simulink model "Trans_model"  (R2020b)
settings: Solver=VariableStepAuto  StartTime=0.0  StopTime=10.0  RelTol=1e-3
libraries: fl_lib x3, nesl_utility x3, ee_lib x2, powerlib_meascontrol x1, simulink x1
settings Model: Creator=1  LastModifiedBy=1

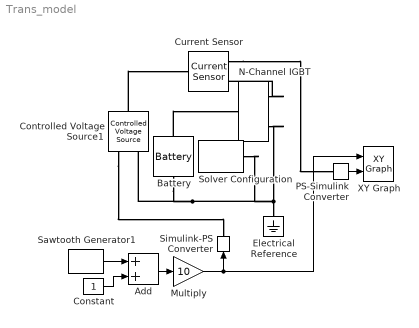
== system Trans_model ==
  Add : Sum
  Battery : ee_lib/Sources/Battery  Vnom=15 V  prm_dir=1  R1_dis=2 Ohm  R1_ch=2 Ohm  R1=1 Ohm  prm_AH=1  AH=50 hr*A  V1=11.5 V  AH1=25 hr*A  prm_R2=1  R2=2000 Ohm  prm_dyn=1  Rp1=0.005 Ohm  tau1=30 s  Rp2=0.005 Ohm  tau2=30 s  Rp3=0.005 Ohm  tau3=30 s  Rp4=0.005 Ohm  tau4=30 s  Rp5=0.005 Ohm  tau5=30 s  prm_fade=1  N_fade=100  AH_fade=45 hr*A  R1_fade=2.02 Ohm  R1_ch_fade=2.02 Ohm  V1_fade=10.35 V  i_specify=off  i_priority=None  i=0 A  i_nominal_specify=off  i_nominal_unit=A  i_nominal_value=1  v_specify=off  v_priority=Low  v=6 V  v_nominal_specify=off  v_nominal_unit=V  v_nominal_value=1  charge_specify=off  charge_priority=High  charge=50 hr*A  charge_nominal_specify=off  charge_nominal_unit=hr*A  charge_nominal_value=1  num_cycles_specify=off  num_cycles_priority=High  num_cycles=0  num_cycles_nominal_specify=off  num_cycles_nominal_unit=1  num_cycles_nominal_value=1  thermal_mass=30000 J/K  Tmeas=298.15 K  Vnom_T2=12 V  R1_T2=2.2 Ohm  R1_T2_dis=2.2 Ohm  R1_T2_ch=2.2 Ohm  V1_T2=11.4 V  R2_T2=2200 Ohm  Rp1_T2=0.005 Ohm  tau1_T2=30 s  Rp2_T2=0.005 Ohm  tau2_T2=30 s  Rp3_T2=0.005 Ohm  tau3_T2=30 s  Rp4_T2=0.005 Ohm  tau4_T2=30 s  Rp5_T2=0.005 Ohm  tau5_T2=30 s  Tmeas2=273.15 K  temperature_specify=off  temperature_priority=High  temperature=298.15 K  temperature_nominal_specify=off  temperature_nominal_unit=K  temperature_nominal_value=1
  Constant : Constant
  Controlled Voltage Source1 : fl_lib/Electrical/Electrical Sources/Controlled Voltage Source
  Current Sensor : fl_lib/Electrical/Electrical Sensors/Current Sensor
  Electrical Reference : fl_lib/Electrical/Electrical Elements/Electrical Reference
  Multiply : Gain  Gain=10
  N-Channel IGBT : ee_lib/Semiconductors & Converters/N-Channel IGBT  model_type=1  Ices=25 uA  Vces=1200 V  Vth=5 V  Vce_sat=3.2 V  Ice_sat=120 A  Vge_sat=15 V  ec=1  Tmeas=110 degC  Vge_vec=[-1, 0, .5, 1, 1.5, 2, 2.5, 3, 3.5, 4] V  Vce_vec=[-2, 6, 7, 8, 10, 12, 15, 20] V  T_vec=[25, 125] degC  Ic_mat=[-1.015e-05, -9.9869e-06, -9.955e-06, -9.955e-06, -9.955e-06, -9.9549e-06, -9.9549e-06, -9.9549e-06; 1.35e-08, 1.35e-08, 1.35e-08, 1.35e-08, 1.35e-08, 1.35e-08, 1.35e-08, 1.35e-08; .00047135, .00047135, .0065225, .0065235, .006524, .0065242, .0065243, .0065244; .0005092, .0005092, 3.3324, 3.5783, 3.7206, 3.7716, 3.8067, 3.8324; .0005105, .0005105, 48.154, 70.264, 89.171, 97.793, 104.52, 109.92; .00051175, .00051175, 93.661, 166.33, 228.09, 256.21, 278.11, 295.67; .00051299, .00051299, 105.52, 252.4, 371.63, 424.27, 464.6, 496.54; .00051423, .00051423, 105.72, 317.67, 511.02, 592.92, 654.37, 702.28; .00051548, .00051548, 105.93, 353.38, 642.69, 759.2, 844.57, 909.96; .00051672, .00051672, 106.14, 357.39, 764.04, 921.52, 1033.9, 1118.3] A  Ic_mat_3D=zeros(10, 8, 2) A  C_param=3  C_GE=23.7 nF  C_GC=2.7 nF  C_CE=0 nF  C_ies=9.85 nF  C_res=0.218 nF  C_oes=0.58 nF  C_GE_vec=[25, 31, 26.5, 24.9, 25, 24.9, 24.6, 24.7, 24.8] nF  C_GC_vec=[55, 9, 5.5, 3.1, 2.5, 2.1, 1.9, 1.8, 1.7] nF  C_CE_vec=[5, 11, 6.5, 4.9, 3.5, 2.7, 2.1, 1.7, 1.4] nF  C_ies_vec=[18, 13, 12, 11, 10, 10, 10, 10, 10] nF  C_res_vec=[6, 2.7, 1.9, 1.3, 0.36, 0.22, 0.19, 0.175, 0.16] nF  C_oes_vec=[8.5, 4, 3, 2, 0.8, 0.6, 0.5, 0.48, 0.43] nF  C_Vce_vec=[0, 5, 10, 15, 20, 25, 30, 35, 40] V  charge_linearity_param=1  C_OX=212 pF  V_C_OX=-5 V  TF=30 ns  VAF=20 V  RC=0.0001 Ohm  RE=0.00005 Ohm  RG=0.001 Ohm  BF=100  T_param=2  Ices_T2=1.5 mA  EG=1.11 eV  Vce_sat_T2=3.4 V  Tmeas2=150 degC  XTI=1  BEX=0  RG_alpha=0 1/K  Tdevice=25 degC  Tdevice_3D=25 degC  thermal_network_parameterization=ee.enum.thermalNetworkTopology.cauer  Rth=[0, 10] K/W  Rth_Foster=[4, 6] K/W  thermal_mass_parameterization=ee.enum.thermalNetwork.timeconstant  thermal_mass=[0, 1] J/K  thermal_mass_Foster=[1.5, 3] J/K  thermal_time_constant=[0, 10] s  thermal_time_constant_Foster=[6, 18] s  thermal_mass_initial_temperatures=[25, 25] degC  Ic_vec1=[0, 10, 50, 100, 200, 400, 600] A  Vce_vec1=[0, 1.1, 1.3, 1.45, 1.75, 2.25, 2.7] V  Rmiller=0.1 Ohm  Goff=1e-5 1/Ohm  t_on=0.07 us  t_rise=0.7 us  t_off=0.2 us  t_fall=0.5 us  v_meas=300 V  Tj_vec1=[298.15, 398.15] K  Vce_mat1=[0, 1.1, 1.3, 1.45, 1.75, 2.25, 2.7; 0, 1, 1.15, 1.35, 1.7, 2.35, 3] V  E_turn_on_mat1=[0, .2, 1, 2, 4, 8, 15; 0, .3, 1.3, 2.5, 5, 11, 18] * 1e-3 J  E_turn_off_mat1=[0, .3, 1.5, 3, 6, 15, 25; 0, .7, 3.3, 6.5, 13, 25, 35] * 1e-3 J
      settings: SourceProductBaseCode=PS  InternalSimscapePortConfiguration="{\"Bottom\":[],\"Left\":[{\"id\":\"G\",\"label\":\"\",\"type\":\"foundation.electrical.electrical\"}],\"Right\":[{\"id\":\"C\",\"label\":\"\",\"type\":\"foundation.electrical.electrical\"},{\"id\":\"E\",\"label\":\"\",\"type\":\"foundation.electrical.electrical\"}],\"Top\":[]}"
  PS-Simulink Converter : nesl_utility/PS-Simulink Converter  PhysicalDomain=network_engine_domain  SubClassName=ps_output  LeftPortType=input  RightPortType=output  PseudoPeriodic=off  Frequencies=[]  Unit=A  AffineConversion=off
  Sawtooth Generator1 : powerlib_meascontrol/Pulse & Signal Generators/Sawtooth Generator  Freq=1e-1  Phase=0  Ts=0
  Simulink-PS Converter : nesl_utility/Simulink-PS Converter  PhysicalDomain=network_engine_domain  SubClassName=ps_input  LeftPortType=input  RightPortType=output  PseudoPeriodic=off  Frequencies=[]  NoiseDistribution=none  NoiseParameters=[]  Unit=V  AffineConversion=off  FilteringAndDerivatives=provide  SimscapeFilterOrder=1  InputFilterTimeConstant=0.001  UdotUserProvided=0
  Solver Configuration : nesl_utility/Solver Configuration  PhysicalDomain=network_engine_domain  SubClassName=solver  LeftPortType=input  RightPortType=generic  Tones=[]  Harmonics=[]  SimulateNoise=off  Profile=off  UseLocalSampling=off  EnableSwitchedLinearOptims=on  FrequencyDomain=off  UseCCode=off  RelTol=0.001  AbsTol=1e-06  MinStep=1e-09  ToWorkspace=off  RevertToSquareIcSolve=off  NumHomotopyIterations=100  PhasorMode=off  PhasorModeNumHarmonics=1  DoDC=off  ResidualTolerance=1e-09  UseLocalSolver=off  LocalSolverChoice=NE_BACKWARD_EULER_ADVANCER  LocalSolverSampleTime=0.001  DoFixedCost=off  MaxNonlinIter=3  MaxModeIter=2  ComputeImpulses=on  ImpulseIterations=2  LinearAlgebra=auto  EquationFormulation=NE_TIME_EF  DelaysMemoryBudget=1024  AutomaticFiltering=on  FilteringTimeConstant=0.00001  PartitionStorageMethod=AS_NEEDED  PartitionMemoryBudget=1024  PartitionMethod=ROBUST
  XY Graph : simulink/Sinks/XY Graph  xmin=0  xmax=4  ymin=0  ymax=160  st=-1
  wires:
  Sawtooth Generator1/1 -> Add/1
  Add/1 -> Multiply/1
  Constant/1 -> Add/2
  Multiply/1 -> Simulink-PS Converter/1, XY Graph/1
  PS-Simulink Converter/1 -> XY Graph/2
  connections:
  N-Channel IGBT/RConn2 -- Solver Configuration/RConn1 -- Controlled Voltage Source1/RConn2 -- Battery/RConn1 -- Electrical Reference/LConn1
  Battery/LConn1 -- N-Channel IGBT/LConn1
  N-Channel IGBT/RConn1 -- Current Sensor/RConn2
  Controlled Voltage Source1/LConn1 -- Current Sensor/LConn1
  Current Sensor/RConn1 -- PS-Simulink Converter/LConn1
  Controlled Voltage Source1/RConn1 -- Simulink-PS Converter/RConn1
